simulink model "Regenerative_braking"  (R2023b)
settings: Solver=VariableStepAuto  StartTime=0.0  StopTime=10.0  RelTol=1e-3
libraries: spsIdealSwitchLib x2, spsACVoltageSourceLib x1, spsSeriesRLCBranchLib x1, spsSinglePhaseAsynchronousMachineLib x1, spspowerguiLib x1
settings Model: Creator=vivek  LastModifiedBy=vivek

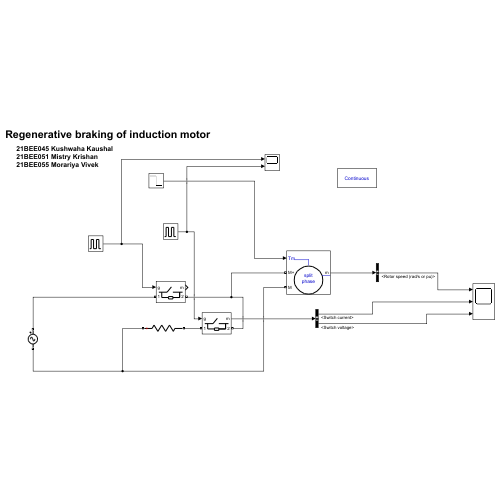
[thumbnail: Simulink's stored preview of the top-level diagram]
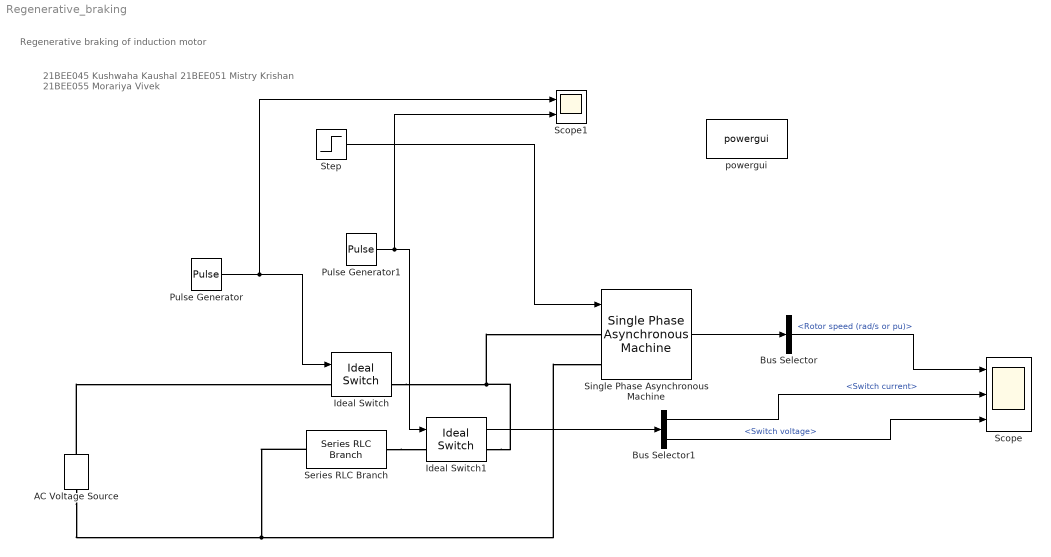
== system Regenerative_braking ==
  note: 21BEE045 Kushwaha Kaushal
      | 21BEE051 Mistry Krishan
      | 21BEE055 Morariya Vivek
  note: Regenerative braking of induction motor
  AC Voltage Source : spsACVoltageSourceLib/AC Voltage Source  Amplitude=600  Phase=0  Frequency=50  SampleTime=0  Measurements=None  BusType=swing  Pref=10e3  Qref=0  Qmin=-inf  Qmax=+inf
  Bus Selector : BusSelector  OutputSignals=Mechanical.Rotor speed (rad/s or pu)
  Bus Selector1 : BusSelector  OutputSignals=Switch current,Switch voltage
  Ideal Switch : spsIdealSwitchLib/Ideal Switch  Ron=0.001  Lon=0  IC=0  Rs=1e5  Cs=inf  Measurements=on
  Ideal Switch1 : spsIdealSwitchLib/Ideal Switch  Ron=0.001  Lon=0  IC=1  Rs=1e5  Cs=inf  Measurements=on
  Pulse Generator : DiscretePulseGenerator  PulseType=Time based  Period=10  PulseWidth=50  PhaseDelay=0.000005
  Pulse Generator1 : DiscretePulseGenerator  PulseType=Time based  Period=10  PulseWidth=50  PhaseDelay=5
  Scope : Scope  NumInputPorts=3
  Scope1 : Scope  NumInputPorts=2
  Series RLC Branch : spsSeriesRLCBranchLib/Series RLC Branch  LConnTagsString=__new0  RConnTagsString=__new0  BranchType=R  Resistance=10  Inductance=1e-3  SetiL0=off  InitialCurrent=0  Capacitance=1e-6  Setx0=off  InitialVoltage=0  Measurements=None
  Single Phase Asynchronous Machine : spsSinglePhaseAsynchronousMachineLib/Single Phase Asynchronous Machine  MechanicalLoad=Torque Tm  UNITS=SI  MachineType=Split Phase  MeasurementBus=off  NominalParameters="[ .25*746  110  50]"  MainWindingStator="[2.02  7.4e-3]"  MainWindingRotor="[4.12  5.6e-3]"  MutualInductance=0.1772  AuxiliaryWinding="[7.14  8.5e-3]"  Mechanical="[0.0132  0.01  2 1.18]"  CapacitorStart="[2  254.7e-6]"  CapacitorRun="[18  21.1e-6]"  DisconnectionSpeed=75  InitialSpeed=0  DataType=SI  TsPowergui=0  TsBlock=-1
      settings: LibrarySourceBlock=|
      | sps_lib/Electrical Machines/Single Phase
      | Asynchronous Machine
  Step : Step  Time=5  Before=1  After=0  SampleTime=0
  powergui : spspowerguiLib/powergui  Priority=1  SimulationMode=Continuous  SampleTime=50e-6  frequency=60  Iterations=50  frequencyindice=50  Pbase=100e6  ErrMax=1e-4  UnitsV=kV  UnitsW=MW  buscounter=0  FunctionMessages=off  echomessages=off  EnableUseOfTLC=off  CurrentSourceSwitches=off  DisableSnubberDevices=off  DisableRonSwitches=off  DisableVfSwitches=off  DisplayEquations=off  AutomaticDiscreteSolvers=off  SolverType=Tustin/Backward Euler (TBE)  Interpol=off  ExternalGateDelay=off  methode=off  Ts=100  x0status=blocks  SPID=on  SwTol=0  HookPort=off  NonlinearTolerance=1e-4  nMaxIteration=100  ContinueOnMaxIteration=off  RestoreLinks=warning  ResistiveCurrentMeasurement=off  Frange=[0:2:500]  Ylog=off  Xlog=on  ShowGrid=off  save=off  variable=ZData  structure=0  ZoomFFT=off  StartTime=0.0  cycles=1  DisplayStyle=1  fundamental=60  FreqAxis=off  MaxFrequency=1000  frequencyindicesteady=1  RmsSteady=1  display=off
  wires:
  Single Phase Asynchronous Machine/1 -> Bus Selector/1
  Bus Selector/1 -> Scope/1  "<Rotor speed (rad/s or pu)>"
  Pulse Generator/1 -> Scope1/1, Ideal Switch/1
  Pulse Generator1/1 -> Scope1/2, Ideal Switch1/1
  Step/1 -> Single Phase Asynchronous Machine/1
  Ideal Switch1/1 -> Bus Selector1/1
  Bus Selector1/1 -> Scope/2  "<Switch current>"
  Bus Selector1/2 -> Scope/3  "<Switch voltage>"
  connections:
  Ideal Switch/RConn1 -- Ideal Switch1/RConn1 -- Single Phase Asynchronous Machine/LConn1
  Series RLC Branch/RConn1 -- Ideal Switch1/LConn1
  AC Voltage Source/LConn1 -- Series RLC Branch/LConn1 -- Single Phase Asynchronous Machine/LConn2
  AC Voltage Source/RConn1 -- Ideal Switch/LConn1
